simulink model "example_SolarCollector1xN"  (R2018b)
settings: Solver=ode45  StartTime=0.0  StopTime=2*24*3600  MaxStep=1800  RelTol=1e-3  EnableMultiTasking=on
libraries: carnot x8
settings Model: Creator=drhf  LastModifiedBy=drhf
settings DataIOCC: LimitDataPoints=on  SaveFormat=Array
settings OptimizationCC: ExpressionDepthLimit=2147483647  LifeSpan=inf
settings DebuggingCC: UnderspecifiedInitializationDetection=Classic  MergeDetectMultiDrivingBlocksExec=none  SolverPrmCheckMsg=warning  StateNameClashWarn=warning  SFUnexpectedBacktrackingDiag=warning  SFNoUnconditionalDefaultTransitionDiag=warning  SFExecutionAtInitializationDiag=none
settings HardwareCC: ProdBitPerPointer=32  ProdBitPerSizeT=32  ProdBitPerPtrDiffT=32  ProdLargestAtomicFloat=None  ProdIntDivRoundTo=Undefined  ProdEndianess=Unspecified  ProdWordSize=32  ProdHWDeviceType=32-bit Generic
settings ModelReferenceCC: PropagateSignalLabelsOutOfModel=off
settings SFSimCC: SimUseLocalCustomCode=off
settings RTWCC: RTWUseLocalCustomCode=off
settings CodeAppCC: StateflowObjectComments=on
settings GRTTargetCC: TargetLangStandard=C89/C90 (ANSI)  GeneratePreprocessorConditionals=Disable all  CombineOutputUpdateFcns=off  GRTInterface=on
settings ConfigComp: CovMetricSettings=dw  CovHtmlReporting=on  CovSaveCumulativeToWorkspaceVar=on  CovSaveSingleToWorkspaceVar=on  CovExternalEMLEnable=off

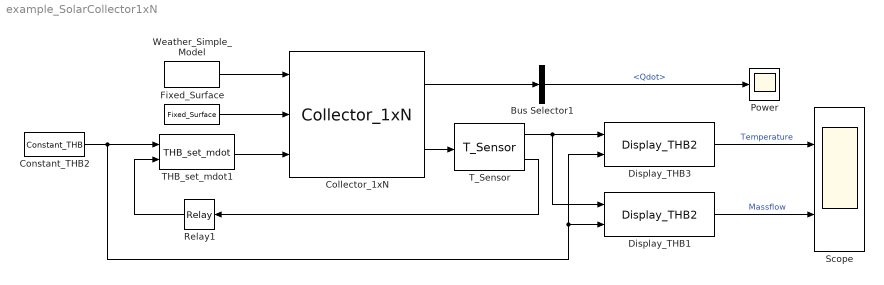
== system example_SolarCollector1xN ==
  Bus Selector1 : BusSelector  OutputSignals=Qdot
  Collector_1xN : carnot/Source/Solar_Thermal/Collector_1xN  acol=2.3  len=2  eta0=0.8  u1=3.5  u2=0.02  u3=0  uwind=0  c_col=1e4  lin=10  qua=10  tini=20  nodes=5
      settings: SourceProductName=Carnot
  Constant_THB2 : carnot/Source/Simple/Constant_THB  t=40  mdot=100/3600  p=1e5  mID=No Pressure Drop  fluid=Water  mix=0  mix2=0  mix3=0  dia=0.02  hgt=0
      settings: SourceProductName=Carnot
  Display_THB1 : carnot/Outputs/Display_THB2  t=off  m=off  p=on  id=off  mix=off  d=off
      settings: SourceProductName=Carnot
  Display_THB3 : carnot/Outputs/Display_THB2  t=off  m=off  p=on  id=off  mix=off  d=off
      settings: SourceProductName=Carnot
  Fixed_Surface : carnot/Weather/Fixed_Surface  colangle=30  colazi=0  colrot=0
      settings: SourceProductName=Carnot
  Power : Scope
  Relay1 : Relay  OnSwitchValue=47  OffSwitchValue=42  OnOutputValue=50/3600
  Scope : Scope  NumInputPorts=2
  THB_set_mdot1 : carnot/Source/Simple/THB_set_mdot
      settings: SourceProductName=Carnot
  T_Sensor : carnot/Control/T_Sensor  tc=10  t0=20
      settings: SourceProductName=Carnot
  Weather_Simple_Model : carnot/Weather/Weather_Simple_Model  lat=60  Ibn=900  Idg=100  tamb=5  deltaTsky=-6  rh=50  precip="10e-3/24/3600           % 10 mm in 24 h"  cloud=0.125  p=1013e2  vw=1  wdir=270
      settings: SourceProductName=Carnot
  wires:
  Weather_Simple_Model/1 -> Collector_1xN/1
  Fixed_Surface/1 -> Collector_1xN/2
  Display_THB3/1 -> Scope/1  "Temperature"
  Collector_1xN/1 -> Bus Selector1/1
  Bus Selector1/1 -> Power/1  "<Qdot>"
  Constant_THB2/1 -> Display_THB1/2, Display_THB3/2, THB_set_mdot1/1
  THB_set_mdot1/1 -> Collector_1xN/3
  T_Sensor/2 -> Relay1/1
  Relay1/1 -> THB_set_mdot1/2
  Display_THB1/1 -> Scope/2  "Massflow"
  T_Sensor/1 -> Display_THB1/1, Display_THB3/1
  Collector_1xN/2 -> T_Sensor/1
